simulink library "motion"  (Simulink 10.0)
settings: Solver=VariableStepAuto  StartTime=0.0  StopTime=10.0  RelTol=1e-3
undefined symbols (not defined in the file): ad, dd, jd
libraries: $bdroot x1
settings Model: Creator=Kamran  LastModifiedBy=Kamran

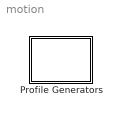
== system motion ==
  Profile Generators : Subsystem
      mask Display: disp('Profile\nGenerators')

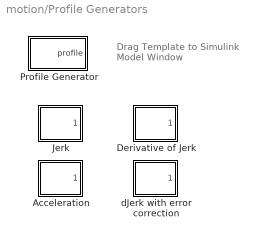
== system motion/Profile Generators ==
  note: Drag Template to
      | Simulink Model Window
  Acceleration : Subsystem  mask(2nd Order Profile Generator){t0=.3, x=1, v=1, a=5, Ts=0}
      mask prompts: t0 "Starting time:  t0 [s]"; x "Displacement:  x [m]"; v "Bound on velocity:  vmax [m/s]"; a "Bound on acceleration:  amax [m/s2]"; Ts "Sampling time (0 for continuous):  Ts [s]"
      mask help: 2nd Order Profile Generator
      mask init:
      | [t,ad,aa,tx,a,v,p,tt] = make2(abs(x),v,a,Ts,0);
      | t0=t0-10*eps;
      mask Help: See make2.m and look under mask
      mask Display:
      | plot([0 aa(1,:)+t0],[0 aa(2,:)])
      | text(0.8*(max(aa(1,:))+t0),0,'a\n')
  Derivative of Jerk : Subsystem  AncestorBlock=library/Derivative of jerk profile generator  mask(4th Order Profile Generator){t0=.3, x=1, v=1, a=5, j=50, d=1000, Ts=0}
      mask prompts: t0 "Starting time:  t0 [s]"; x "Displacement:  x [m]"; v "Bound on velocity:  vmax [m/s]"; a "Bound on acceleration:  amax [m/s2]"; j "Bound on jerk: jmax [m/s3]"; d "Bound on derivative of jerk:  dmax [m/s4]"; Ts "Sampling time (0 for continuous):  Ts [s]"
      mask help: 4th Order Profile Generator
      mask init:
      | [t,dd]=make4(abs(x),v,a,j,d,Ts);
      | t0=t0-10*eps;
      | [dj,tx,d,j,a,v,p,tt]=profile4(t,dd(1),0,0);
      mask Help: See make4.m and profile4.m and look under mask
      mask Display:
      | plot([0 dj(1,:)+t0],[0 dj(2,:)])
      | text(0.8*(max(dj(1,:))+t0),0,'d\n')
  Jerk : Subsystem  mask(3d Order Profile Generator){t0=.3, x=1, v=1, a=5, j=50, Ts=0}
      mask prompts: t0 "Starting time:  t0 [s]"; x "Displacement:  x [m]"; v "Bound on velocity:  vmax [m/s]"; a "Bound on acceleration:  amax [m/s2]"; j "Bound on jerk: jmax [m/s3]"; Ts "Sampling time (0 for continuous):  Ts [s]"
      mask help: 3d Order Profile Generator
      mask init:
      | [t,jd]=make3(abs(x),v,a,j,Ts);
      | t0=t0-10*eps;
      | [jj,tx,j,a,v,p,tt]=profile3(t,jd(1),0,0);
      mask Help: See make3.m and profile3.m and look under mask
      mask Display:
      | plot([0 jj(1,:)+t0],[0 jj(2,:)])
      | text(0.85*(max(jj(1,:))+t0),0,'j\n')
  Profile Generator : Subsystem  BlockChoice=Acceleration
      settings: TemplateBlock=self  MemberBlocks=Acceleration,Derivative of Jerk,Jerk,dJerk with error correction
  dJerk with error correction : Subsystem  mask(4th Order Profile Generator with quantization error correction){t0=.3, x=1, v=1, a=5, j=50, d=1000, Ts=0, r=10*eps, s=15}
      mask prompts: t0 "Starting time:  t0 [s]"; x "Displacement:  x [m]"; v "Bound on velocity:  vmax [m/s]"; a "Bound on acceleration:  amax [m/s2]"; j "Bound on jerk: jmax [m/s3]"; d "Bound on derivative of jerk:  dmax [m/s4]"; Ts "Sampling time (0 for continuous):  Ts [s]"; r "Resolution of position [m] (default: 10*eps)"; s "Number of decimals for digitized d (default: 15)"
      mask help: 4th Order Profile Generator with quantization error correction
      mask init:
      | if length(r)==0 | length(s)==0
      | 	r=10*eps;
      | 	s=15;
      | end
      | [t,dd]=make4(abs(x),v,a,j,d,Ts,r,s);
      | t0=t0-10*eps;
      | [dj,tx,d,j,a,v,p,tt]=profile4(t,dd(1),0,0);
      mask Help: See make4.m and profile4.m and look under mask
      mask Display:
      | plot([0 dj(1,:)+t0],[0 dj(2,:)])
      | text(0.8*(max(dj(1,:))+t0),0,'d\n')

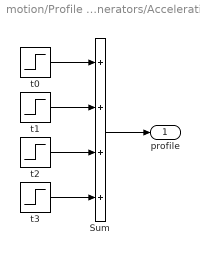
== system motion/Profile Generators/Acceleration ==
  Sum : Sum  Inputs=4  SaturateOnIntegerOverflow=on  InputSameDT=on  OutDataTypeStr=Inherit: Same as first input
  t0 : Step  Time=t0  After=ad(1)  SampleTime=0
  t1 : Step  Time=t0+t(1)  After=-ad(1)  SampleTime=0
  t2 : Step  Time=t0+t(1)+t(2)  After=-ad(1)  SampleTime=0
  t3 : Step  Time=t0+2*t(1)+t(2)  After=ad(1)  SampleTime=0
  profile : Outport
  wires:
  t0/1 -> Sum/1
  t1/1 -> Sum/2
  t2/1 -> Sum/3
  t3/1 -> Sum/4
  Sum/1 -> profile/1

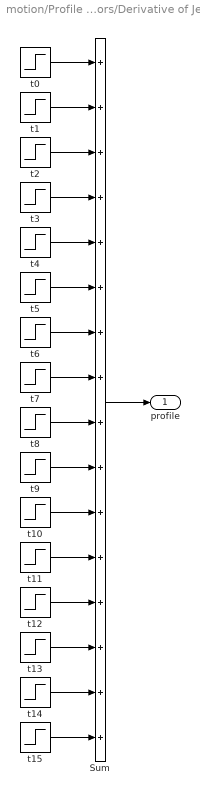
== system motion/Profile Generators/Derivative of Jerk ==
  Sum : Sum  Inputs=16  SaturateOnIntegerOverflow=on  InputSameDT=on  OutDataTypeStr=Inherit: Same as first input
  t0 : Step  Time=t0  After=dd(1)  SampleTime=0
  t1 : Step  Time=t0+t(1)  After=-dd(1)  SampleTime=0
  t10 : Step  Time=t0+5*t(1)+3*t(2)+t(3)+t(4)  After=dd(1)  SampleTime=0
  t11 : Step  Time=t0+6*t(1)+3*t(2)+t(3)+t(4)  After=-dd(1)  SampleTime=0
  t12 : Step  Time=t0+6*t(1)+3*t(2)+2*t(3)+t(4)  After=dd(1)  SampleTime=0
  t13 : Step  Time=t0+7*t(1)+3*t(2)+2*t(3)+t(4)  After=-dd(1)  SampleTime=0
  t14 : Step  Time=t0+7*t(1)+4*t(2)+2*t(3)+t(4)  After=-dd(1)  SampleTime=0
  t15 : Step  Time=t0+8*t(1)+4*t(2)+2*t(3)+t(4)  After=dd(1)  SampleTime=0
  t2 : Step  Time=t0+t(1)+t(2)  After=-dd(1)  SampleTime=0
  t3 : Step  Time=t0+2*t(1)+t(2)  After=dd(1)  SampleTime=0
  t4 : Step  Time=t0+2*t(1)+t(2)+t(3)  After=-dd(1)  SampleTime=0
  t5 : Step  Time=t0+3*t(1)+t(2)+t(3)  After=dd(1)  SampleTime=0
  t6 : Step  Time=t0+3*t(1)+2*t(2)+t(3)  After=dd(1)  SampleTime=0
  t7 : Step  Time=t0+4*t(1)+2*t(2)+t(3)  After=-dd(1)  SampleTime=0
  t8 : Step  Time=t0+4*t(1)+2*t(2)+t(3)+t(4)  After=-dd(1)  SampleTime=0
  t9 : Step  Time=t0+5*t(1)+2*t(2)+t(3)+t(4)  After=dd(1)  SampleTime=0
  profile : Outport
  wires:
  t0/1 -> Sum/1
  t1/1 -> Sum/2
  t2/1 -> Sum/3
  t3/1 -> Sum/4
  t4/1 -> Sum/5
  t5/1 -> Sum/6
  t6/1 -> Sum/7
  t7/1 -> Sum/8
  t8/1 -> Sum/9
  t9/1 -> Sum/10
  t10/1 -> Sum/11
  t11/1 -> Sum/12
  t12/1 -> Sum/13
  t13/1 -> Sum/14
  t14/1 -> Sum/15
  t15/1 -> Sum/16
  Sum/1 -> profile/1

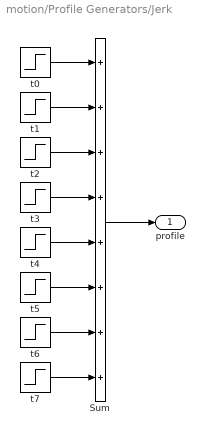
== system motion/Profile Generators/Jerk ==
  Sum : Sum  Inputs=8  SaturateOnIntegerOverflow=on  InputSameDT=on  OutDataTypeStr=Inherit: Same as first input
  t0 : Step  Time=t0  After=jd(1)  SampleTime=0
  t1 : Step  Time=t0+t(1)  After=-jd(1)  SampleTime=0
  t2 : Step  Time=t0+t(1)+t(2)  After=-jd(1)  SampleTime=0
  t3 : Step  Time=t0+2*t(1)+t(2)  After=jd(1)  SampleTime=0
  t4 : Step  Time=t0+2*t(1)+t(2)+t(3)  After=-jd(1)  SampleTime=0
  t5 : Step  Time=t0+3*t(1)+t(2)+t(3)  After=jd(1)  SampleTime=0
  t6 : Step  Time=t0+3*t(1)+2*t(2)+t(3)  After=jd(1)  SampleTime=0
  t7 : Step  Time=t0+4*t(1)+2*t(2)+t(3)  After=-jd(1)  SampleTime=0
  profile : Outport
  wires:
  Sum/1 -> profile/1
  t7/1 -> Sum/8
  t6/1 -> Sum/7
  t5/1 -> Sum/6
  t4/1 -> Sum/5
  t3/1 -> Sum/4
  t2/1 -> Sum/3
  t1/1 -> Sum/2
  t0/1 -> Sum/1

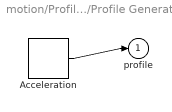
== system motion/Profile Generators/Profile Generator ==
  Acceleration : $bdroot/Profile Generators/Acceleration  t0=.3  x=1  v=1  a=5  Ts=0
  profile : Outport
  wires:
  Acceleration/1 -> profile/1

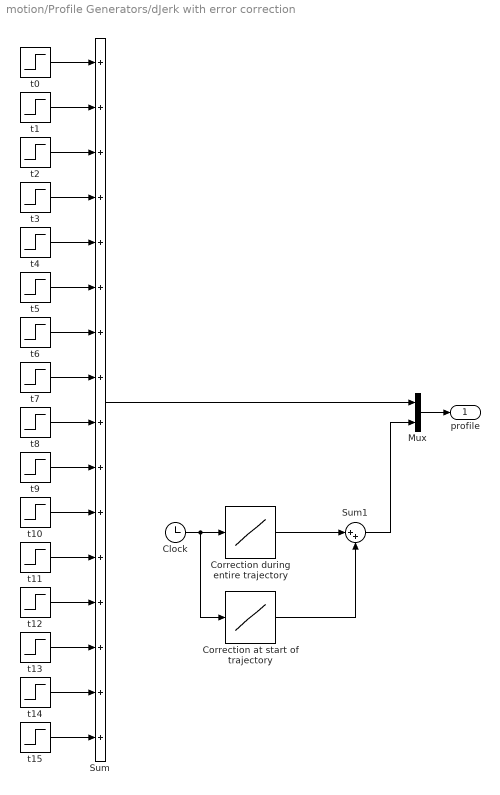
== system motion/Profile Generators/dJerk with error correction ==
  Clock : Clock
  Correction at start of trajectory : Lookup  InputValues="[ -1 t0 t0+abs(dd(3))*Ts  2*(t0+8*t(1)+4*t(2)+2*t(3)+t(4)) ]"  Table=[ 0 0 [1 1]*dd(3)*r]  SaturateOnIntegerOverflow=on
  Correction during entire trajectory : Lookup  InputValues="[ -1 t0  t0+8*t(1)+4*t(2)+2*t(3)+t(4)  2*(t0+8*t(1)+4*t(2)+2*t(3)+t(4)) ]"  Table=[0 0 [1 1]*dd(2)*r]  SaturateOnIntegerOverflow=on
  Mux : Mux  Inputs=2
  Sum : Sum  Inputs=16  SaturateOnIntegerOverflow=on  InputSameDT=on  OutDataTypeStr=Inherit: Same as first input
  Sum1 : Sum  Inputs=|++  SaturateOnIntegerOverflow=on  InputSameDT=on  OutDataTypeStr=Inherit: Same as first input
  t0 : Step  Time=t0  After=dd(1)  SampleTime=0
  t1 : Step  Time=t0+t(1)  After=-dd(1)  SampleTime=0
  t10 : Step  Time=t0+5*t(1)+3*t(2)+t(3)+t(4)  After=dd(1)  SampleTime=0
  t11 : Step  Time=t0+6*t(1)+3*t(2)+t(3)+t(4)  After=-dd(1)  SampleTime=0
  t12 : Step  Time=t0+6*t(1)+3*t(2)+2*t(3)+t(4)  After=dd(1)  SampleTime=0
  t13 : Step  Time=t0+7*t(1)+3*t(2)+2*t(3)+t(4)  After=-dd(1)  SampleTime=0
  t14 : Step  Time=t0+7*t(1)+4*t(2)+2*t(3)+t(4)  After=-dd(1)  SampleTime=0
  t15 : Step  Time=t0+8*t(1)+4*t(2)+2*t(3)+t(4)  After=dd(1)  SampleTime=0
  t2 : Step  Time=t0+t(1)+t(2)  After=-dd(1)  SampleTime=0
  t3 : Step  Time=t0+2*t(1)+t(2)  After=dd(1)  SampleTime=0
  t4 : Step  Time=t0+2*t(1)+t(2)+t(3)  After=-dd(1)  SampleTime=0
  t5 : Step  Time=t0+3*t(1)+t(2)+t(3)  After=dd(1)  SampleTime=0
  t6 : Step  Time=t0+3*t(1)+2*t(2)+t(3)  After=dd(1)  SampleTime=0
  t7 : Step  Time=t0+4*t(1)+2*t(2)+t(3)  After=-dd(1)  SampleTime=0
  t8 : Step  Time=t0+4*t(1)+2*t(2)+t(3)+t(4)  After=-dd(1)  SampleTime=0
  t9 : Step  Time=t0+5*t(1)+2*t(2)+t(3)+t(4)  After=dd(1)  SampleTime=0
  profile : Outport
  wires:
  Sum/1 -> Mux/1
  Mux/1 -> profile/1
  t0/1 -> Sum/1
  t1/1 -> Sum/2
  t2/1 -> Sum/3
  t3/1 -> Sum/4
  t4/1 -> Sum/5
  t5/1 -> Sum/6
  t6/1 -> Sum/7
  t7/1 -> Sum/8
  t8/1 -> Sum/9
  t9/1 -> Sum/10
  t10/1 -> Sum/11
  t11/1 -> Sum/12
  t12/1 -> Sum/13
  t13/1 -> Sum/14
  t14/1 -> Sum/15
  t15/1 -> Sum/16
  Clock/1 -> Correction during entire trajectory/1, Correction at start of trajectory/1
  Correction at start of trajectory/1 -> Sum1/2
  Sum1/1 -> Mux/2
  Correction during entire trajectory/1 -> Sum1/1
